simulink model "MRACSISO"  (R2022a)
settings: Solver=FixedStepAuto  StartTime=0.0  StopTime=3000.0  FixedStep=0.001  RelTol=1e-3
libraries: cstblocks x2
settings Model: Creator=loryb  LastModifiedBy=loryb

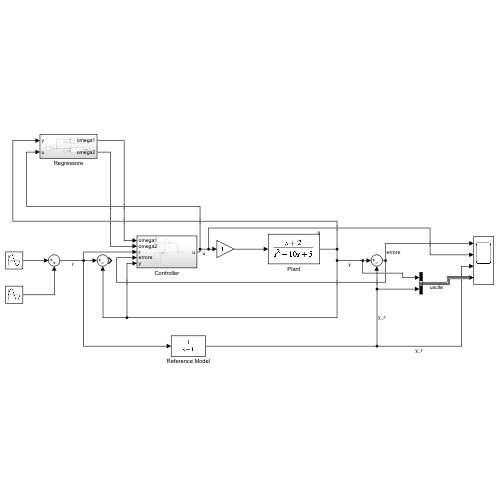
[thumbnail: Simulink's stored preview of the top-level diagram]
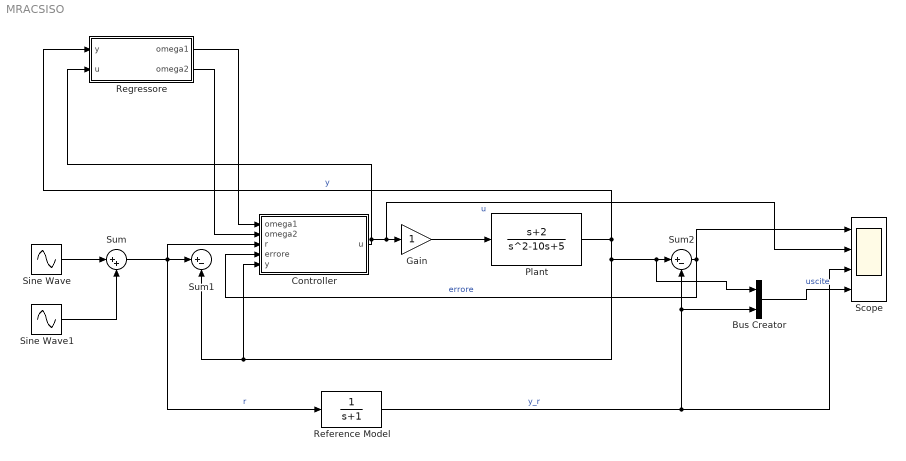
== system MRACSISO ==
  Bus Creator : BusCreator  Inputs=2
  Controller : Subsystem
  Gain : Gain
  Plant : TransferFcn  Numerator=[1 2]  Denominator=[1 -10 5]
  Reference Model : TransferFcn  Denominator=[1 1]
  Regressore : Subsystem
  Scope : Scope  NumInputPorts=4
  Sine Wave : Sin  Frequency=5  SampleTime=0
  Sine Wave1 : Sin  SampleTime=0
  Sum : Sum  Inputs=|++
  Sum1 : Sum  Inputs=|+-
  Sum2 : Sum  Inputs=|+-
  wires:
  Gain/1 -> Plant/1
  Sine Wave/1 -> Sum/1
  Sine Wave1/1 -> Sum/2
  Sum/1 -> Reference Model/1, Sum1/1, Controller/3(r)  "r"
  Controller/1(u) -> Scope/2, Gain/1, Regressore/2(u)  "u"
  Plant/1 -> Bus Creator/1, Sum2/1, Sum1/2, Controller/5(y), Regressore/1(y)  "y"
  Reference Model/1 -> Scope/3, Bus Creator/2, Sum2/2  "y_r"
  Sum2/1 -> Controller/4(errore), Scope/1  "errore"
  Regressore/1(omega1) -> Controller/1(omega1)
  Regressore/2(omega2) -> Controller/2(omega2)
  Bus Creator/1 -> Scope/4  "uscite"

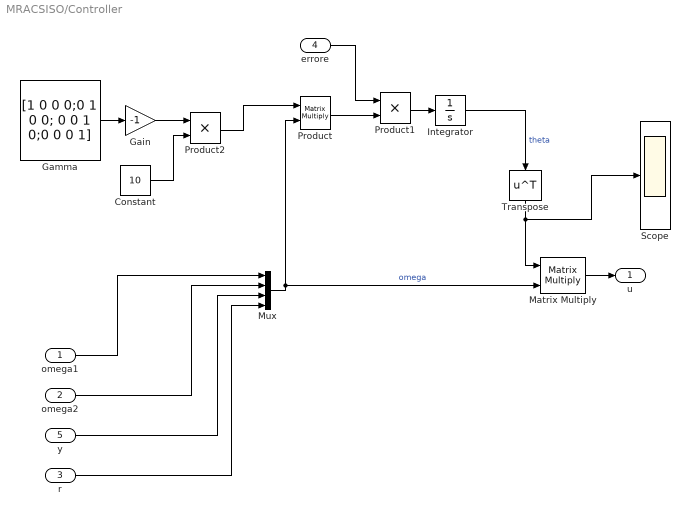
== system MRACSISO/Controller ==
  omega1 : Inport
  omega2 : Inport  Port=2
  r : Inport  Port=3
  errore : Inport  Port=4
  y : Inport  Port=5
  Constant : Constant  Value=10
  Gain : Gain  Gain=-1
  Gamma : Constant  Value=[1 0 0 0;0 1 0 0; 0 0 1 0;0 0 0 1]  VectorParams1D=off
  Integrator : Integrator
  Matrix Multiply : Product  Multiplication=Matrix(*)
  Mux : Mux
  Product : Product  Multiplication=Matrix(*)
  Product1 : Product
  Product2 : Product
  Scope : Scope
  Transpose : Math  Operator=transpose
  u : Outport
  wires:
  omega1/1 -> Mux/1
  omega2/1 -> Mux/2
  y/1 -> Mux/3
  r/1 -> Mux/4
  Gamma/1 -> Gain/1
  Product/1 -> Product1/2
  Integrator/1 -> Transpose/1  "theta"
  errore/1 -> Product1/1
  Product1/1 -> Integrator/1
  Mux/1 -> Matrix Multiply/2, Product/2  "omega"
  Transpose/1 -> Scope/1, Matrix Multiply/1
  Matrix Multiply/1 -> u/1
  Gain/1 -> Product2/1
  Product2/1 -> Product/1
  Constant/1 -> Product2/2

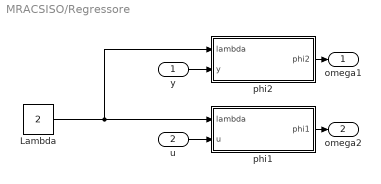
== system MRACSISO/Regressore ==
  y : Inport
  u : Inport  Port=2
  Lambda : Constant  Value=2
  phi1 : Subsystem
  phi2 : Subsystem
  omega1 : Outport
  omega2 : Outport  Port=2
  wires:
  Lambda/1 -> phi1/1(lambda), phi2/1(lambda)
  u/1 -> phi1/2(u)
  y/1 -> phi2/2(y)
  phi1/1(phi1) -> omega2/1
  phi2/1(phi2) -> omega1/1

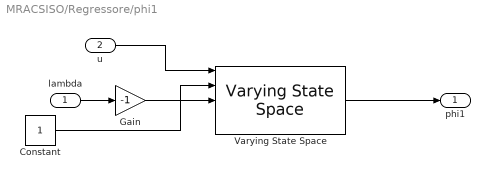
== system MRACSISO/Regressore/phi1 ==
  lambda : Inport
  u : Inport  Port=2
  Constant : Constant
  Gain : Gain  Gain=-1
  Varying State Space : cstblocks/Linear Parameter Varying/Varying State Space  x0=0  xNames=''  OutputX=on  OutputDX=on
  phi1 : Outport
  wires:
  lambda/1 -> Gain/1
  u/1 -> Varying State Space/1
  Gain/1 -> Varying State Space/2
  Constant/1 -> Varying State Space/3
  Varying State Space/2 -> phi1/1

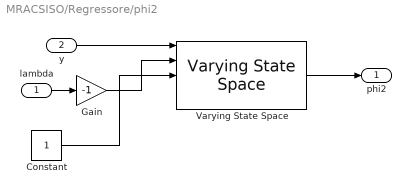
== system MRACSISO/Regressore/phi2 ==
  lambda : Inport
  y : Inport  Port=2
  Constant : Constant
  Gain : Gain  Gain=-1
  Varying State Space : cstblocks/Linear Parameter Varying/Varying State Space  x0=0  xNames=''  OutputX=on  OutputDX=on
  phi2 : Outport
  wires:
  lambda/1 -> Gain/1
  y/1 -> Varying State Space/1
  Gain/1 -> Varying State Space/2
  Constant/1 -> Varying State Space/3
  Varying State Space/2 -> phi2/1
